simulink model "Saturation_verif"  (Simulink 7.2)
settings: Solver=ode45  StartTime=0.0  StopTime=10.0  RelTol=1e-3
undefined symbols (not defined in the file): sample
settings Model: Creator=Romain  LastModifiedBy=Romain
settings OptimizationCC: ExpressionDepthLimit=128
settings DebuggingCC: SolverPrmCheckMsg=none  FcnCallInpInsideContextMsg=Enable All  StateNameClashWarn=none  StrictBusMsg=ErrorLevel1
settings CodeAppCC: CustomSymbolStrType=$N$R$M_T
settings GRTTargetCC: TargetFunctionLibrary=C89/C90 (ANSI)

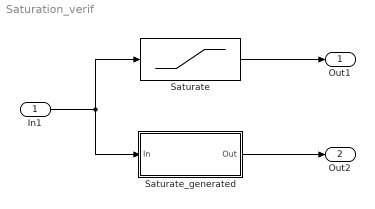
== system Saturation_verif ==
  In1 : Inport  OutDataTypeStr=double  DataType=double
  Saturate : Saturate
  Saturate_generated : Subsystem  TreatAsAtomicUnit=on
  Out1 : Outport
  Out2 : Outport  Port=2
  wires:
  In1/1 -> Saturate_generated/1(In), Saturate/1
  Saturate/1 -> Out1/1
  Saturate_generated/1(Out) -> Out2/1

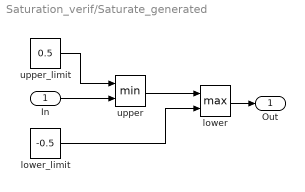
== system Saturation_verif/Saturate_generated ==
  In : Inport
  lower : MinMax  Function=max  Inputs=2
  lower_limit : Constant  Value=-0.5  SampleTime=sample
  upper : MinMax  Inputs=2
  upper_limit : Constant  Value=0.5  SampleTime=sample
  Out : Outport
  wires:
  upper_limit/1 -> upper/1
  upper/1 -> lower/1
  lower_limit/1 -> lower/2
  In/1 -> upper/2
  lower/1 -> Out/1
